simulink model "EPT"  (R2019b)
settings: Solver=FixedStepDiscrete  StartTime=0.0  StopTime=5  FixedStep=0.005  RelTol=1e-3  EnableMultiTasking=on
PreLoadFcn:
  | try, model_open; catch, disp('Error occurred while executing model pre-load callback: model_open.m'); disp('Please assure that the MATLAB working directory is set to the model directory before opening.'); end
InitFcn:
  | try, model_open; catch, end
undefined symbols (not defined in the file or in its folder): Bridge, GCM, H, ln, raptor_get_param_eval, raptor_get_safe_string, raptor_xcp_function
libraries: Raptor_lib x2810, simulink x374, hdlsllib x19
(part 36 of 45)

== system EPT/Foreground_TimeBase_5ms/E//W /BP-OBU_E//W/BP-OBU_E//W/BP-OBU_Warning//Fault_G5/Latch43 ==
  Latch : Inport
  Reset : Inport  Port=2
  Switch1 : Switch  Criteria=u2 > Threshold
  Switch3 : Switch  Criteria=u2 > Threshold
  Unit Delay1 : UnitDelay  SampleTime=-1  HasFrameUpgradeWarning=on
  Output : Outport  VectorParamsAs1DForOutWhenUnconnected=off
  wires:
  Unit Delay1/1 -> Switch1/3
  Switch3/1 -> Output/1, Unit Delay1/1
  Reset/1 -> Switch3/2
  Latch/1 -> Switch1/1, Switch1/2
  Switch1/1 -> Switch3/3

== system EPT/Foreground_TimeBase_5ms/E//W /BP-OBU_E//W/BP-OBU_E//W/BP-OBU_Warning//Fault_G5/Latch44 ==
  Latch : Inport
  Reset : Inport  Port=2
  Switch1 : Switch  Criteria=u2 > Threshold
  Switch3 : Switch  Criteria=u2 > Threshold
  Unit Delay1 : UnitDelay  SampleTime=-1  HasFrameUpgradeWarning=on
  Output : Outport  VectorParamsAs1DForOutWhenUnconnected=off
  wires:
  Switch1/1 -> Switch3/3
  Latch/1 -> Switch1/2, Switch1/1
  Reset/1 -> Switch3/2
  Switch3/1 -> Unit Delay1/1, Output/1
  Unit Delay1/1 -> Switch1/3

== system EPT/Foreground_TimeBase_5ms/E//W /BP-OBU_E//W/BP-OBU_E//W/BP-OBU_Warning//Fault_G5/Latch45 ==
  Latch : Inport
  Reset : Inport  Port=2
  Switch1 : Switch  Criteria=u2 > Threshold
  Switch3 : Switch  Criteria=u2 > Threshold
  Unit Delay1 : UnitDelay  SampleTime=-1  HasFrameUpgradeWarning=on
  Output : Outport  VectorParamsAs1DForOutWhenUnconnected=off
  wires:
  Unit Delay1/1 -> Switch1/3
  Switch3/1 -> Output/1, Unit Delay1/1
  Reset/1 -> Switch3/2
  Latch/1 -> Switch1/1, Switch1/2
  Switch1/1 -> Switch3/3

== system EPT/Foreground_TimeBase_5ms/E//W /BP-OBU_E//W/BP-OBU_E//W/BP-OBU_Warning//Fault_G5/Latch46 ==
  Latch : Inport
  Reset : Inport  Port=2
  Switch1 : Switch  Criteria=u2 > Threshold
  Switch3 : Switch  Criteria=u2 > Threshold
  Unit Delay1 : UnitDelay  SampleTime=-1  HasFrameUpgradeWarning=on
  Output : Outport  VectorParamsAs1DForOutWhenUnconnected=off
  wires:
  Switch1/1 -> Switch3/3
  Latch/1 -> Switch1/2, Switch1/1
  Reset/1 -> Switch3/2
  Switch3/1 -> Unit Delay1/1, Output/1
  Unit Delay1/1 -> Switch1/3

== system EPT/Foreground_TimeBase_5ms/E//W /BP-OBU_E//W/BP-OBU_E//W/BP-OBU_Warning//Fault_G5/Latch47 ==
  Latch : Inport
  Reset : Inport  Port=2
  Switch1 : Switch  Criteria=u2 > Threshold
  Switch3 : Switch  Criteria=u2 > Threshold
  Unit Delay1 : UnitDelay  SampleTime=-1  HasFrameUpgradeWarning=on
  Output : Outport  VectorParamsAs1DForOutWhenUnconnected=off
  wires:
  Unit Delay1/1 -> Switch1/3
  Switch3/1 -> Output/1, Unit Delay1/1
  Reset/1 -> Switch3/2
  Latch/1 -> Switch1/1, Switch1/2
  Switch1/1 -> Switch3/3

== system EPT/Foreground_TimeBase_5ms/E//W /BP-OBU_E//W/BP-OBU_E//W/BP-OBU_Warning//Fault_G5/Latch48 ==
  Latch : Inport
  Reset : Inport  Port=2
  Switch1 : Switch  Criteria=u2 > Threshold
  Switch3 : Switch  Criteria=u2 > Threshold
  Unit Delay1 : UnitDelay  SampleTime=-1  HasFrameUpgradeWarning=on
  Output : Outport  VectorParamsAs1DForOutWhenUnconnected=off
  wires:
  Switch1/1 -> Switch3/3
  Latch/1 -> Switch1/2, Switch1/1
  Reset/1 -> Switch3/2
  Switch3/1 -> Unit Delay1/1, Output/1
  Unit Delay1/1 -> Switch1/3

== system EPT/Foreground_TimeBase_5ms/E//W /BP-OBU_E//W/BP-OBU_E//W/BP-OBU_Warning//Fault_G5/Latch49 ==
  Latch : Inport
  Reset : Inport  Port=2
  Switch1 : Switch  Criteria=u2 > Threshold
  Switch3 : Switch  Criteria=u2 > Threshold
  Unit Delay1 : UnitDelay  SampleTime=-1  HasFrameUpgradeWarning=on
  Output : Outport  VectorParamsAs1DForOutWhenUnconnected=off
  wires:
  Unit Delay1/1 -> Switch1/3
  Switch3/1 -> Output/1, Unit Delay1/1
  Reset/1 -> Switch3/2
  Latch/1 -> Switch1/1, Switch1/2
  Switch1/1 -> Switch3/3

== system EPT/Foreground_TimeBase_5ms/E//W /CAN_E//W/CAN_Fault/BCU CAN Fault/BCU LifeCycle Fault ==
  note: CMU_All_20ms LifeCycle
  note: CMU_All_200ms LifeCycle
  Reset : Inport
  OBC Work : Inport  Port=2
  If Action Subsystem10 : Subsystem  TreatAsAtomicUnit=on
  If Action Subsystem11 : Subsystem  TreatAsAtomicUnit=on
  If Action Subsystem12 : Subsystem  TreatAsAtomicUnit=on
  If Action Subsystem13 : Subsystem  TreatAsAtomicUnit=on
  If Action Subsystem18 : Subsystem  TreatAsAtomicUnit=on
  If Action Subsystem9 : Subsystem  TreatAsAtomicUnit=on
  Latch10 : Subsystem
  Latch11 : Subsystem
  Latch12 : Subsystem
  Latch13 : Subsystem
  Latch14 : Subsystem
  Latch19 : Subsystem
  raptor_data_def1 : Raptor_lib/Data Storage/raptor_data_def  dataName='LifeCycle_Fault_CMU200B0A2'  initValue=0  dataType=boolean  storage=Volatile (RAM)  calVisible=on  calType=Measurement  calDispType=Number  calEnum={'False', 'True'}  calGain=1.0  calOffset=0  calMin=-inf  calMax=inf  calFormat='-1'  calUnit=''  calHelp=''  calAccess=1  calFunction=raptor_xcp_function(gcb)  calDispHeaders=off  calColHeaders={'Col1' 'Col2' 'Col3'}  calRowHeaders={'Row1' 'Row2' 'Row3'}
      settings: SourceProductName=Raptor
  raptor_data_def2 : Raptor_lib/Data Storage/raptor_data_def  dataName='LifeCycle_Fault_CMU200B1A1'  initValue=0  dataType=boolean  storage=Volatile (RAM)  calVisible=on  calType=Measurement  calDispType=Number  calEnum={'False', 'True'}  calGain=1.0  calOffset=0  calMin=-inf  calMax=inf  calFormat='-1'  calUnit=''  calHelp=''  calAccess=1  calFunction=raptor_xcp_function(gcb)  calDispHeaders=off  calColHeaders={'Col1' 'Col2' 'Col3'}  calRowHeaders={'Row1' 'Row2' 'Row3'}
      settings: SourceProductName=Raptor
  raptor_data_def3 : Raptor_lib/Data Storage/raptor_data_def  dataName='LifeCycle_Fault_CMU200B1A2'  initValue=0  dataType=boolean  storage=Volatile (RAM)  calVisible=on  calType=Measurement  calDispType=Number  calEnum={'False', 'True'}  calGain=1.0  calOffset=0  calMin=-inf  calMax=inf  calFormat='-1'  calUnit=''  calHelp=''  calAccess=1  calFunction=raptor_xcp_function(gcb)  calDispHeaders=off  calColHeaders={'Col1' 'Col2' 'Col3'}  calRowHeaders={'Row1' 'Row2' 'Row3'}
      settings: SourceProductName=Raptor
  raptor_data_def31 : Raptor_lib/Data Storage/raptor_data_def  dataName='Flag_B2_200ms'  initValue=0  dataType=boolean  storage=Volatile (RAM)  calVisible=on  calType=Measurement  calDispType=Number  calEnum={'False', 'True'}  calGain=1.0  calOffset=0  calMin=-inf  calMax=inf  calFormat='-1'  calUnit=''  calHelp=''  calAccess=1  calFunction=raptor_xcp_function(gcb)  calDispHeaders=off  calColHeaders={'Col1' 'Col2' 'Col3'}  calRowHeaders={'Row1' 'Row2' 'Row3'}
      settings: SourceProductName=Raptor
  raptor_data_def39 : Raptor_lib/Data Storage/raptor_data_def  dataName='Flag_B0_B1_20ms'  initValue=0  dataType=boolean  storage=Volatile (RAM)  calVisible=on  calType=Measurement  calDispType=Number  calEnum={'False', 'True'}  calGain=1.0  calOffset=0  calMin=-inf  calMax=inf  calFormat='-1'  calUnit=''  calHelp=''  calAccess=1  calFunction=raptor_xcp_function(gcb)  calDispHeaders=off  calColHeaders={'Col1' 'Col2' 'Col3'}  calRowHeaders={'Row1' 'Row2' 'Row3'}
      settings: SourceProductName=Raptor
  raptor_data_def4 : Raptor_lib/Data Storage/raptor_data_def  dataName='LifeCycle_Fault_CMU200B2A1'  initValue=0  dataType=boolean  storage=Volatile (RAM)  calVisible=on  calType=Measurement  calDispType=Number  calEnum={'False', 'True'}  calGain=1.0  calOffset=0  calMin=-inf  calMax=inf  calFormat='-1'  calUnit=''  calHelp=''  calAccess=1  calFunction=raptor_xcp_function(gcb)  calDispHeaders=off  calColHeaders={'Col1' 'Col2' 'Col3'}  calRowHeaders={'Row1' 'Row2' 'Row3'}
      settings: SourceProductName=Raptor
  raptor_data_def5 : Raptor_lib/Data Storage/raptor_data_def  dataName='LifeCycle_Fault_CMU200B2A2'  initValue=0  dataType=boolean  storage=Volatile (RAM)  calVisible=on  calType=Measurement  calDispType=Number  calEnum={'False', 'True'}  calGain=1.0  calOffset=0  calMin=-inf  calMax=inf  calFormat='-1'  calUnit=''  calHelp=''  calAccess=1  calFunction=raptor_xcp_function(gcb)  calDispHeaders=off  calColHeaders={'Col1' 'Col2' 'Col3'}  calRowHeaders={'Row1' 'Row2' 'Row3'}
      settings: SourceProductName=Raptor
  raptor_data_def8 : Raptor_lib/Data Storage/raptor_data_def  dataName='LifeCycle_Fault_CMU200B0A1'  initValue=0  dataType=boolean  storage=Volatile (RAM)  calVisible=on  calType=Measurement  calDispType=Number  calEnum={'False', 'True'}  calGain=1.0  calOffset=0  calMin=-inf  calMax=inf  calFormat='-1'  calUnit=''  calHelp=''  calAccess=1  calFunction=raptor_xcp_function(gcb)  calDispHeaders=off  calColHeaders={'Col1' 'Col2' 'Col3'}  calRowHeaders={'Row1' 'Row2' 'Row3'}
      settings: SourceProductName=Raptor
  raptor_data_read29 : Raptor_lib/Data Storage/raptor_data_read  dataName='CMU1_B0_RC'  dataShape=Scalar  idxSource=Input  idxRow=1  idxCol=1
      settings: SourceProductName=Raptor
  raptor_data_read32 : Raptor_lib/Data Storage/raptor_data_read  dataName='CMU2_B0_RC'  dataShape=Scalar  idxSource=Input  idxRow=1  idxCol=1
      settings: SourceProductName=Raptor
  raptor_data_read33 : Raptor_lib/Data Storage/raptor_data_read  dataName='CMU1_B1_RC'  dataShape=Scalar  idxSource=Input  idxRow=1  idxCol=1
      settings: SourceProductName=Raptor
  raptor_data_read34 : Raptor_lib/Data Storage/raptor_data_read  dataName='CMU1_B2_RC'  dataShape=Scalar  idxSource=Input  idxRow=1  idxCol=1
      settings: SourceProductName=Raptor
  raptor_data_read35 : Raptor_lib/Data Storage/raptor_data_read  dataName='CMU2_B2_RC'  dataShape=Scalar  idxSource=Input  idxRow=1  idxCol=1
      settings: SourceProductName=Raptor
  raptor_data_read41 : Raptor_lib/Data Storage/raptor_data_read  dataName='CMU2_B1_RC'  dataShape=Scalar  idxSource=Input  idxRow=1  idxCol=1
      settings: SourceProductName=Raptor
  raptor_data_read42 : Raptor_lib/Data Storage/raptor_data_read  dataName='Flag_B0_B1_20ms'  dataShape=Scalar  idxSource=Input  idxRow=1  idxCol=1
      settings: SourceProductName=Raptor
  raptor_data_read43 : Raptor_lib/Data Storage/raptor_data_read  dataName='Flag_B2_200ms'  dataShape=Scalar  idxSource=Input  idxRow=1  idxCol=1
      settings: SourceProductName=Raptor
  raptor_data_write23 : Raptor_lib/Data Storage/raptor_data_write  dataName='LifeCycle_Fault_CMU200B0A1'  dataShape=Scalar  idxSource=Input Port  idxRow=1  idxCol=1
      settings: SourceProductName=Raptor
  raptor_data_write24 : Raptor_lib/Data Storage/raptor_data_write  dataName='LifeCycle_Fault_CMU200B0A2'  dataShape=Scalar  idxSource=Input Port  idxRow=1  idxCol=1
      settings: SourceProductName=Raptor
  raptor_data_write25 : Raptor_lib/Data Storage/raptor_data_write  dataName='LifeCycle_Fault_CMU200B1A1'  dataShape=Scalar  idxSource=Input Port  idxRow=1  idxCol=1
      settings: SourceProductName=Raptor
  raptor_data_write26 : Raptor_lib/Data Storage/raptor_data_write  dataName='LifeCycle_Fault_CMU200B2A1'  dataShape=Scalar  idxSource=Input Port  idxRow=1  idxCol=1
      settings: SourceProductName=Raptor
  raptor_data_write27 : Raptor_lib/Data Storage/raptor_data_write  dataName='LifeCycle_Fault_CMU200B2A2'  dataShape=Scalar  idxSource=Input Port  idxRow=1  idxCol=1
      settings: SourceProductName=Raptor
  raptor_data_write32 : Raptor_lib/Data Storage/raptor_data_write  dataName='LifeCycle_Fault_CMU200B1A2'  dataShape=Scalar  idxSource=Input Port  idxRow=1  idxCol=1
      settings: SourceProductName=Raptor
  wires:
  raptor_data_read41/1 -> If Action Subsystem18/1(LifeCycle)
  Latch11/1(Output) -> raptor_data_write25/1
  Latch10/1(Output) -> raptor_data_write23/1
  If Action Subsystem13/1(Trigger) -> Latch14/1(Latch)
  Latch12/1(Output) -> raptor_data_write24/1
  If Action Subsystem18/1(Trigger) -> Latch19/1(Latch)
  raptor_data_read32/1 -> If Action Subsystem11/1(LifeCycle)
  raptor_data_read29/1 -> If Action Subsystem10/1(LifeCycle)
  If Action Subsystem9/1(Trigger) -> Latch11/1(Latch)
  raptor_data_read33/1 -> If Action Subsystem9/1(LifeCycle)
  raptor_data_read43/1 -> If Action Subsystem13/Enable, If Action Subsystem12/Enable
  Reset/1 -> Latch10/2(Reset), Latch19/2(Reset), Latch13/2(Reset), Latch14/2(Reset), Latch11/2(Reset), Latch12/2(Reset)
  raptor_data_read34/1 -> If Action Subsystem12/1(LifeCycle)
  Latch19/1(Output) -> raptor_data_write32/1
  OBC Work/1 -> If Action Subsystem13/2(CanWork), If Action Subsystem12/2(CanWork), If Action Subsystem18/2(CanWork), If Action Subsystem9/2(CanWork), If Action Subsystem11/2(CanWork), If Action Subsystem10/2(CanWork)
  If Action Subsystem10/1(Trigger) -> Latch10/1(Latch)
  raptor_data_read35/1 -> If Action Subsystem13/1(LifeCycle)
  Latch14/1(Output) -> raptor_data_write27/1
  Latch13/1(Output) -> raptor_data_write26/1
  If Action Subsystem11/1(Trigger) -> Latch12/1(Latch)
  If Action Subsystem12/1(Trigger) -> Latch13/1(Latch)
  raptor_data_read42/1 -> If Action Subsystem10/Enable, If Action Subsystem18/Enable, If Action Subsystem9/Enable, If Action Subsystem11/Enable

== system EPT/Foreground_TimeBase_5ms/E//W /CAN_E//W/CAN_Fault/BCU CAN Fault/Error10 ==
  Condition : Inport
  Reset : Inport  Port=2
  Constant : Constant  Value=boolean('1')
  NOT : Logic  Operator=NOT  IconShape=distinctive  AllPortsSameDT=off  OutDataTypeStr=boolean
  Switch : Switch  Criteria=u2 > Threshold
  Switch12 : Switch  Criteria=u2 > Threshold
  Unit Delay : UnitDelay  SampleTime=-1  HasFrameUpgradeWarning=on
  Error : Outport  VectorParamsAs1DForOutWhenUnconnected=off
  wires:
  Constant/1 -> Switch/1, NOT/1
  Unit Delay/1 -> Switch/3
  Switch/1 -> Switch12/3
  Switch12/1 -> Unit Delay/1, Error/1
  Condition/1 -> Switch/2
  Reset/1 -> Switch12/2
  NOT/1 -> Switch12/1

== system EPT/Foreground_TimeBase_5ms/E//W /CAN_E//W/CAN_Fault/BCU CAN Fault/Error11 ==
  Condition : Inport
  Reset : Inport  Port=2
  Constant : Constant  Value=boolean('1')
  NOT : Logic  Operator=NOT  IconShape=distinctive  AllPortsSameDT=off  OutDataTypeStr=boolean
  Switch : Switch  Criteria=u2 > Threshold
  Switch12 : Switch  Criteria=u2 > Threshold
  Unit Delay : UnitDelay  SampleTime=-1  HasFrameUpgradeWarning=on
  Error : Outport  VectorParamsAs1DForOutWhenUnconnected=off
  wires:
  NOT/1 -> Switch12/1
  Reset/1 -> Switch12/2
  Condition/1 -> Switch/2
  Switch12/1 -> Error/1, Unit Delay/1
  Switch/1 -> Switch12/3
  Unit Delay/1 -> Switch/3
  Constant/1 -> NOT/1, Switch/1

== system EPT/Foreground_TimeBase_5ms/E//W /CAN_E//W/CAN_Fault/BCU CAN Fault/Error12 ==
  Condition : Inport
  Reset : Inport  Port=2
  Constant : Constant  Value=boolean('1')
  NOT : Logic  Operator=NOT  IconShape=distinctive  AllPortsSameDT=off  OutDataTypeStr=boolean
  Switch : Switch  Criteria=u2 > Threshold
  Switch12 : Switch  Criteria=u2 > Threshold
  Unit Delay : UnitDelay  SampleTime=-1  HasFrameUpgradeWarning=on
  Error : Outport  VectorParamsAs1DForOutWhenUnconnected=off
  wires:
  Constant/1 -> Switch/1, NOT/1
  Unit Delay/1 -> Switch/3
  Switch/1 -> Switch12/3
  Switch12/1 -> Unit Delay/1, Error/1
  Condition/1 -> Switch/2
  Reset/1 -> Switch12/2
  NOT/1 -> Switch12/1

== system EPT/Foreground_TimeBase_5ms/E//W /CAN_E//W/CAN_Fault/BCU CAN Fault/Error13 ==
  Condition : Inport
  Reset : Inport  Port=2
  Constant : Constant  Value=boolean('1')
  NOT : Logic  Operator=NOT  IconShape=distinctive  AllPortsSameDT=off  OutDataTypeStr=boolean
  Switch : Switch  Criteria=u2 > Threshold
  Switch12 : Switch  Criteria=u2 > Threshold
  Unit Delay : UnitDelay  SampleTime=-1  HasFrameUpgradeWarning=on
  Error : Outport  VectorParamsAs1DForOutWhenUnconnected=off
  wires:
  NOT/1 -> Switch12/1
  Reset/1 -> Switch12/2
  Condition/1 -> Switch/2
  Switch12/1 -> Error/1, Unit Delay/1
  Switch/1 -> Switch12/3
  Unit Delay/1 -> Switch/3
  Constant/1 -> NOT/1, Switch/1

== system EPT/Foreground_TimeBase_5ms/E//W /CAN_E//W/CAN_Fault/BCU CAN Fault/Error3 ==
  Condition : Inport
  Reset : Inport  Port=2
  Constant : Constant  Value=boolean('1')
  NOT : Logic  Operator=NOT  IconShape=distinctive  AllPortsSameDT=off  OutDataTypeStr=boolean
  Switch : Switch  Criteria=u2 > Threshold
  Switch12 : Switch  Criteria=u2 > Threshold
  Unit Delay : UnitDelay  SampleTime=-1  HasFrameUpgradeWarning=on
  Error : Outport  VectorParamsAs1DForOutWhenUnconnected=off
  wires:
  NOT/1 -> Switch12/1
  Reset/1 -> Switch12/2
  Condition/1 -> Switch/2
  Switch12/1 -> Error/1, Unit Delay/1
  Switch/1 -> Switch12/3
  Unit Delay/1 -> Switch/3
  Constant/1 -> NOT/1, Switch/1

== system EPT/Foreground_TimeBase_5ms/E//W /CAN_E//W/CAN_Fault/BCU CAN Fault/Error4 ==
  Condition : Inport
  Reset : Inport  Port=2
  Constant : Constant  Value=boolean('1')
  NOT : Logic  Operator=NOT  IconShape=distinctive  AllPortsSameDT=off  OutDataTypeStr=boolean
  Switch : Switch  Criteria=u2 > Threshold
  Switch12 : Switch  Criteria=u2 > Threshold
  Unit Delay : UnitDelay  SampleTime=-1  HasFrameUpgradeWarning=on
  Error : Outport  VectorParamsAs1DForOutWhenUnconnected=off
  wires:
  Constant/1 -> Switch/1, NOT/1
  Unit Delay/1 -> Switch/3
  Switch/1 -> Switch12/3
  Switch12/1 -> Unit Delay/1, Error/1
  Condition/1 -> Switch/2
  Reset/1 -> Switch12/2
  NOT/1 -> Switch12/1

== system EPT/Foreground_TimeBase_5ms/E//W /CAN_E//W/CAN_Fault/BCU CAN Fault/Error6 ==
  Condition : Inport
  Reset : Inport  Port=2
  Constant : Constant  Value=boolean('1')
  NOT : Logic  Operator=NOT  IconShape=distinctive  AllPortsSameDT=off  OutDataTypeStr=boolean
  Switch : Switch  Criteria=u2 > Threshold
  Switch12 : Switch  Criteria=u2 > Threshold
  Unit Delay : UnitDelay  SampleTime=-1  HasFrameUpgradeWarning=on
  Error : Outport  VectorParamsAs1DForOutWhenUnconnected=off
  wires:
  NOT/1 -> Switch12/1
  Reset/1 -> Switch12/2
  Condition/1 -> Switch/2
  Switch12/1 -> Error/1, Unit Delay/1
  Switch/1 -> Switch12/3
  Unit Delay/1 -> Switch/3
  Constant/1 -> NOT/1, Switch/1

== system EPT/Foreground_TimeBase_5ms/E//W /CAN_E//W/CAN_Fault/BCU CAN Fault/Error7 ==
  Condition : Inport
  Reset : Inport  Port=2
  Constant : Constant  Value=boolean('1')
  NOT : Logic  Operator=NOT  IconShape=distinctive  AllPortsSameDT=off  OutDataTypeStr=boolean
  Switch : Switch  Criteria=u2 > Threshold
  Switch12 : Switch  Criteria=u2 > Threshold
  Unit Delay : UnitDelay  SampleTime=-1  HasFrameUpgradeWarning=on
  Error : Outport  VectorParamsAs1DForOutWhenUnconnected=off
  wires:
  Constant/1 -> Switch/1, NOT/1
  Unit Delay/1 -> Switch/3
  Switch/1 -> Switch12/3
  Switch12/1 -> Unit Delay/1, Error/1
  Condition/1 -> Switch/2
  Reset/1 -> Switch12/2
  NOT/1 -> Switch12/1

== system EPT/Foreground_TimeBase_5ms/E//W /CAN_E//W/CAN_Fault/BCU CAN Fault/Error8 ==
  Condition : Inport
  Reset : Inport  Port=2
  Constant : Constant  Value=boolean('1')
  NOT : Logic  Operator=NOT  IconShape=distinctive  AllPortsSameDT=off  OutDataTypeStr=boolean
  Switch : Switch  Criteria=u2 > Threshold
  Switch12 : Switch  Criteria=u2 > Threshold
  Unit Delay : UnitDelay  SampleTime=-1  HasFrameUpgradeWarning=on
  Error : Outport  VectorParamsAs1DForOutWhenUnconnected=off
  wires:
  NOT/1 -> Switch12/1
  Reset/1 -> Switch12/2
  Condition/1 -> Switch/2
  Switch12/1 -> Error/1, Unit Delay/1
  Switch/1 -> Switch12/3
  Unit Delay/1 -> Switch/3
  Constant/1 -> NOT/1, Switch/1

== system EPT/Foreground_TimeBase_5ms/E//W /CAN_E//W/CAN_Fault/BCU CAN Fault/Error9 ==
  Condition : Inport
  Reset : Inport  Port=2
  Constant : Constant  Value=boolean('1')
  NOT : Logic  Operator=NOT  IconShape=distinctive  AllPortsSameDT=off  OutDataTypeStr=boolean
  Switch : Switch  Criteria=u2 > Threshold
  Switch12 : Switch  Criteria=u2 > Threshold
  Unit Delay : UnitDelay  SampleTime=-1  HasFrameUpgradeWarning=on
  Error : Outport  VectorParamsAs1DForOutWhenUnconnected=off
  wires:
  Constant/1 -> Switch/1, NOT/1
  Unit Delay/1 -> Switch/3
  Switch/1 -> Switch12/3
  Switch12/1 -> Unit Delay/1, Error/1
  Condition/1 -> Switch/2
  Reset/1 -> Switch12/2
  NOT/1 -> Switch12/1

== system EPT/Foreground_TimeBase_5ms/E//W /CAN_E//W/CAN_Fault/BCU CAN Fault/Latch1 ==
  Latch : Inport
  Reset : Inport  Port=2
  Switch1 : Switch  Criteria=u2 > Threshold
  Switch3 : Switch  Criteria=u2 > Threshold
  Unit Delay1 : UnitDelay  SampleTime=-1  HasFrameUpgradeWarning=on
  Output : Outport  VectorParamsAs1DForOutWhenUnconnected=off
  wires:
  Unit Delay1/1 -> Switch1/3
  Switch3/1 -> Output/1, Unit Delay1/1
  Reset/1 -> Switch3/2
  Latch/1 -> Switch1/1, Switch1/2
  Switch1/1 -> Switch3/3

== system EPT/Foreground_TimeBase_5ms/E//W /CAN_E//W/CAN_Fault/BCU CAN Fault/deBounce 12 ==
  >= : Inport
  TimeCount1 : Inport  Port=2
  Constant10 : Constant
  Constant11 : Constant  Value=0
  Constant8 : Constant  Value=0
  CycleTrigger1 : Subsystem
  Switch2 : Switch  Threshold=1
  Switch3 : Switch  Threshold=1
  Unit Delay2 : UnitDelay  SampleTime=-1  HasFrameUpgradeWarning=on
  Tirgger1 : Outport  VectorParamsAs1DForOutWhenUnconnected=off
  wires:
  Constant11/1 -> Switch3/3
  Switch2/1 -> Switch3/1
  Switch3/1 -> CycleTrigger1/1(In1)
  Constant10/1 -> Switch2/3
  Unit Delay2/1 -> Switch2/2
  Constant8/1 -> Switch2/1
  CycleTrigger1/1(Trigger) -> Tirgger1/1, Unit Delay2/1
  >=/1 -> Switch3/2
  TimeCount1/1 -> CycleTrigger1/2(In2)

== system EPT/Foreground_TimeBase_5ms/E//W /CAN_E//W/CAN_Fault/BCU CAN Fault/deBounce 13 ==
  >= : Inport
  TimeCount1 : Inport  Port=2
  Constant10 : Constant
  Constant11 : Constant  Value=0
  Constant8 : Constant  Value=0
  CycleTrigger1 : Subsystem
  Switch2 : Switch  Threshold=1
  Switch3 : Switch  Threshold=1
  Unit Delay2 : UnitDelay  SampleTime=-1  HasFrameUpgradeWarning=on
  Tirgger1 : Outport  VectorParamsAs1DForOutWhenUnconnected=off
  wires:
  TimeCount1/1 -> CycleTrigger1/2(In2)
  >=/1 -> Switch3/2
  CycleTrigger1/1(Trigger) -> Unit Delay2/1, Tirgger1/1
  Constant8/1 -> Switch2/1
  Unit Delay2/1 -> Switch2/2
  Constant10/1 -> Switch2/3
  Switch3/1 -> CycleTrigger1/1(In1)
  Switch2/1 -> Switch3/1
  Constant11/1 -> Switch3/3

== system EPT/Foreground_TimeBase_5ms/E//W /CAN_E//W/CAN_Fault/BCU CAN Fault/deBounce 14 ==
  >= : Inport
  TimeCount1 : Inport  Port=2
  Constant10 : Constant
  Constant11 : Constant  Value=0
  Constant8 : Constant  Value=0
  CycleTrigger1 : Subsystem
  Switch2 : Switch  Threshold=1
  Switch3 : Switch  Threshold=1
  Unit Delay2 : UnitDelay  SampleTime=-1  HasFrameUpgradeWarning=on
  Tirgger1 : Outport  VectorParamsAs1DForOutWhenUnconnected=off
  wires:
  Constant11/1 -> Switch3/3
  Switch2/1 -> Switch3/1
  Switch3/1 -> CycleTrigger1/1(In1)
  Constant10/1 -> Switch2/3
  Unit Delay2/1 -> Switch2/2
  Constant8/1 -> Switch2/1
  CycleTrigger1/1(Trigger) -> Tirgger1/1, Unit Delay2/1
  >=/1 -> Switch3/2
  TimeCount1/1 -> CycleTrigger1/2(In2)

== system EPT/Foreground_TimeBase_5ms/E//W /CAN_E//W/CAN_Fault/BCU CAN Fault/deBounce 15 ==
  >= : Inport
  TimeCount1 : Inport  Port=2
  Constant10 : Constant
  Constant11 : Constant  Value=0
  Constant8 : Constant  Value=0
  CycleTrigger1 : Subsystem
  Switch2 : Switch  Threshold=1
  Switch3 : Switch  Threshold=1
  Unit Delay2 : UnitDelay  SampleTime=-1  HasFrameUpgradeWarning=on
  Tirgger1 : Outport  VectorParamsAs1DForOutWhenUnconnected=off
  wires:
  TimeCount1/1 -> CycleTrigger1/2(In2)
  >=/1 -> Switch3/2
  CycleTrigger1/1(Trigger) -> Unit Delay2/1, Tirgger1/1
  Constant8/1 -> Switch2/1
  Unit Delay2/1 -> Switch2/2
  Constant10/1 -> Switch2/3
  Switch3/1 -> CycleTrigger1/1(In1)
  Switch2/1 -> Switch3/1
  Constant11/1 -> Switch3/3

== system EPT/Foreground_TimeBase_5ms/E//W /CAN_E//W/CAN_Fault/BCU CAN Fault/deBounce 16 ==
  >= : Inport
  TimeCount1 : Inport  Port=2
  Constant10 : Constant
  Constant11 : Constant  Value=0
  Constant8 : Constant  Value=0
  CycleTrigger1 : Subsystem
  Switch2 : Switch  Threshold=1
  Switch3 : Switch  Threshold=1
  Unit Delay2 : UnitDelay  SampleTime=-1  HasFrameUpgradeWarning=on
  Tirgger1 : Outport  VectorParamsAs1DForOutWhenUnconnected=off
  wires:
  Constant11/1 -> Switch3/3
  Switch2/1 -> Switch3/1
  Switch3/1 -> CycleTrigger1/1(In1)
  Constant10/1 -> Switch2/3
  Unit Delay2/1 -> Switch2/2
  Constant8/1 -> Switch2/1
  CycleTrigger1/1(Trigger) -> Tirgger1/1, Unit Delay2/1
  >=/1 -> Switch3/2
  TimeCount1/1 -> CycleTrigger1/2(In2)

== system EPT/Foreground_TimeBase_5ms/E//W /CAN_E//W/CAN_Fault/BCU CAN Fault/deBounce 4 ==
  >= : Inport
  TimeCount1 : Inport  Port=2
  Constant10 : Constant
  Constant11 : Constant  Value=0
  Constant8 : Constant  Value=0
  CycleTrigger1 : Subsystem
  Switch2 : Switch  Threshold=1
  Switch3 : Switch  Threshold=1
  Unit Delay2 : UnitDelay  SampleTime=-1  HasFrameUpgradeWarning=on
  Tirgger1 : Outport  VectorParamsAs1DForOutWhenUnconnected=off
  wires:
  TimeCount1/1 -> CycleTrigger1/2(In2)
  >=/1 -> Switch3/2
  CycleTrigger1/1(Trigger) -> Unit Delay2/1, Tirgger1/1
  Constant8/1 -> Switch2/1
  Unit Delay2/1 -> Switch2/2
  Constant10/1 -> Switch2/3
  Switch3/1 -> CycleTrigger1/1(In1)
  Switch2/1 -> Switch3/1
  Constant11/1 -> Switch3/3

== system EPT/Foreground_TimeBase_5ms/E//W /CAN_E//W/CAN_Fault/BCU CAN Fault/deBounce 5 ==
  >= : Inport
  TimeCount1 : Inport  Port=2
  Constant10 : Constant
  Constant11 : Constant  Value=0
  Constant8 : Constant  Value=0
  CycleTrigger1 : Subsystem
  Switch2 : Switch  Threshold=1
  Switch3 : Switch  Threshold=1
  Unit Delay2 : UnitDelay  SampleTime=-1  HasFrameUpgradeWarning=on
  Tirgger1 : Outport  VectorParamsAs1DForOutWhenUnconnected=off
  wires:
  Constant11/1 -> Switch3/3
  Switch2/1 -> Switch3/1
  Switch3/1 -> CycleTrigger1/1(In1)
  Constant10/1 -> Switch2/3
  Unit Delay2/1 -> Switch2/2
  Constant8/1 -> Switch2/1
  CycleTrigger1/1(Trigger) -> Tirgger1/1, Unit Delay2/1
  >=/1 -> Switch3/2
  TimeCount1/1 -> CycleTrigger1/2(In2)

== system EPT/Foreground_TimeBase_5ms/E//W /CAN_E//W/CAN_Fault/BCU CAN Fault/deBounce 6 ==
  >= : Inport
  TimeCount1 : Inport  Port=2
  Constant10 : Constant
  Constant11 : Constant  Value=0
  Constant8 : Constant  Value=0
  CycleTrigger1 : Subsystem
  Switch2 : Switch  Threshold=1
  Switch3 : Switch  Threshold=1
  Unit Delay2 : UnitDelay  SampleTime=-1  HasFrameUpgradeWarning=on
  Tirgger1 : Outport  VectorParamsAs1DForOutWhenUnconnected=off
  wires:
  TimeCount1/1 -> CycleTrigger1/2(In2)
  >=/1 -> Switch3/2
  CycleTrigger1/1(Trigger) -> Unit Delay2/1, Tirgger1/1
  Constant8/1 -> Switch2/1
  Unit Delay2/1 -> Switch2/2
  Constant10/1 -> Switch2/3
  Switch3/1 -> CycleTrigger1/1(In1)
  Switch2/1 -> Switch3/1
  Constant11/1 -> Switch3/3

== system EPT/Foreground_TimeBase_5ms/E//W /CAN_E//W/CAN_Fault/BCU CAN Fault/deBounce 7 ==
  >= : Inport
  TimeCount1 : Inport  Port=2
  Constant10 : Constant
  Constant11 : Constant  Value=0
  Constant8 : Constant  Value=0
  CycleTrigger1 : Subsystem
  Switch2 : Switch  Threshold=1
  Switch3 : Switch  Threshold=1
  Unit Delay2 : UnitDelay  SampleTime=-1  HasFrameUpgradeWarning=on
  Tirgger1 : Outport  VectorParamsAs1DForOutWhenUnconnected=off
  wires:
  Constant11/1 -> Switch3/3
  Switch2/1 -> Switch3/1
  Switch3/1 -> CycleTrigger1/1(In1)
  Constant10/1 -> Switch2/3
  Unit Delay2/1 -> Switch2/2
  Constant8/1 -> Switch2/1
  CycleTrigger1/1(Trigger) -> Tirgger1/1, Unit Delay2/1
  >=/1 -> Switch3/2
  TimeCount1/1 -> CycleTrigger1/2(In2)

== system EPT/Foreground_TimeBase_5ms/E//W /CAN_E//W/CAN_Fault/BCU CAN Fault/deBounce 8 ==
  >= : Inport
  TimeCount1 : Inport  Port=2
  Constant10 : Constant
  Constant11 : Constant  Value=0
  Constant8 : Constant  Value=0
  CycleTrigger1 : Subsystem
  Switch2 : Switch  Threshold=1
  Switch3 : Switch  Threshold=1
  Unit Delay2 : UnitDelay  SampleTime=-1  HasFrameUpgradeWarning=on
  Tirgger1 : Outport  VectorParamsAs1DForOutWhenUnconnected=off
  wires:
  TimeCount1/1 -> CycleTrigger1/2(In2)
  >=/1 -> Switch3/2
  CycleTrigger1/1(Trigger) -> Unit Delay2/1, Tirgger1/1
  Constant8/1 -> Switch2/1
  Unit Delay2/1 -> Switch2/2
  Constant10/1 -> Switch2/3
  Switch3/1 -> CycleTrigger1/1(In1)
  Switch2/1 -> Switch3/1
  Constant11/1 -> Switch3/3

== system EPT/Foreground_TimeBase_5ms/E//W /CAN_E//W/CAN_Fault/BCU CAN Fault/deBounce 9 ==
  >= : Inport
  TimeCount1 : Inport  Port=2
  Constant10 : Constant
  Constant11 : Constant  Value=0
  Constant8 : Constant  Value=0
  CycleTrigger1 : Subsystem
  Switch2 : Switch  Threshold=1
  Switch3 : Switch  Threshold=1
  Unit Delay2 : UnitDelay  SampleTime=-1  HasFrameUpgradeWarning=on
  Tirgger1 : Outport  VectorParamsAs1DForOutWhenUnconnected=off
  wires:
  Constant11/1 -> Switch3/3
  Switch2/1 -> Switch3/1
  Switch3/1 -> CycleTrigger1/1(In1)
  Constant10/1 -> Switch2/3
  Unit Delay2/1 -> Switch2/2
  Constant8/1 -> Switch2/1
  CycleTrigger1/1(Trigger) -> Tirgger1/1, Unit Delay2/1
  >=/1 -> Switch3/2
  TimeCount1/1 -> CycleTrigger1/2(In2)

== system EPT/Foreground_TimeBase_5ms/E//W /CAN_E//W/CAN_Fault/DCDC CAN Fault/Latch1 ==
  Latch : Inport
  Reset : Inport  Port=2
  Switch1 : Switch  Criteria=u2 > Threshold
  Switch3 : Switch  Criteria=u2 > Threshold
  Unit Delay1 : UnitDelay  SampleTime=-1  HasFrameUpgradeWarning=on
  Output : Outport  VectorParamsAs1DForOutWhenUnconnected=off
  wires:
  Switch1/1 -> Switch3/3
  Latch/1 -> Switch1/2, Switch1/1
  Reset/1 -> Switch3/2
  Switch3/1 -> Unit Delay1/1, Output/1
  Unit Delay1/1 -> Switch1/3

== system EPT/Foreground_TimeBase_5ms/E//W /CAN_E//W/CAN_Fault/DCDC CAN Fault/Latch2 ==
  Latch : Inport
  Reset : Inport  Port=2
  Switch1 : Switch  Criteria=u2 > Threshold
  Switch3 : Switch  Criteria=u2 > Threshold
  Unit Delay1 : UnitDelay  SampleTime=-1  HasFrameUpgradeWarning=on
  Output : Outport  VectorParamsAs1DForOutWhenUnconnected=off
  wires:
  Unit Delay1/1 -> Switch1/3
  Switch3/1 -> Output/1, Unit Delay1/1
  Reset/1 -> Switch3/2
  Latch/1 -> Switch1/1, Switch1/2
  Switch1/1 -> Switch3/3

== system EPT/Foreground_TimeBase_5ms/E//W /CAN_E//W/CAN_Fault/DCDC CAN Fault/deBounce 1 ==
  >= : Inport
  TimeCount1 : Inport  Port=2
  Constant10 : Constant
  Constant11 : Constant  Value=0
  Constant8 : Constant  Value=0
  CycleTrigger1 : Subsystem
  Switch2 : Switch  Threshold=1
  Switch3 : Switch  Threshold=1
  Unit Delay2 : UnitDelay  SampleTime=-1  HasFrameUpgradeWarning=on
  Tirgger1 : Outport  VectorParamsAs1DForOutWhenUnconnected=off
  wires:
  TimeCount1/1 -> CycleTrigger1/2(In2)
  >=/1 -> Switch3/2
  CycleTrigger1/1(Trigger) -> Unit Delay2/1, Tirgger1/1
  Constant8/1 -> Switch2/1
  Unit Delay2/1 -> Switch2/2
  Constant10/1 -> Switch2/3
  Switch3/1 -> CycleTrigger1/1(In1)
  Switch2/1 -> Switch3/1
  Constant11/1 -> Switch3/3

== system EPT/Foreground_TimeBase_5ms/E//W /CAN_E//W/CAN_Fault/DCDC CAN Fault/deBounce 10 ==
  >= : Inport
  TimeCount1 : Inport  Port=2
  Constant10 : Constant
  Constant11 : Constant  Value=0
  Constant8 : Constant  Value=0
  CycleTrigger1 : Subsystem
  Switch2 : Switch  Threshold=1
  Switch3 : Switch  Threshold=1
  Unit Delay2 : UnitDelay  SampleTime=-1  HasFrameUpgradeWarning=on
  Tirgger1 : Outport  VectorParamsAs1DForOutWhenUnconnected=off
  wires:
  Constant11/1 -> Switch3/3
  Switch2/1 -> Switch3/1
  Switch3/1 -> CycleTrigger1/1(In1)
  Constant10/1 -> Switch2/3
  Unit Delay2/1 -> Switch2/2
  Constant8/1 -> Switch2/1
  CycleTrigger1/1(Trigger) -> Tirgger1/1, Unit Delay2/1
  >=/1 -> Switch3/2
  TimeCount1/1 -> CycleTrigger1/2(In2)

== system EPT/Foreground_TimeBase_5ms/E//W /CAN_E//W/CAN_Fault/ECHS CAN Fault/Latch1 ==
  Latch : Inport
  Reset : Inport  Port=2
  Switch1 : Switch  Criteria=u2 > Threshold
  Switch3 : Switch  Criteria=u2 > Threshold
  Unit Delay1 : UnitDelay  SampleTime=-1  HasFrameUpgradeWarning=on
  Output : Outport  VectorParamsAs1DForOutWhenUnconnected=off
  wires:
  Unit Delay1/1 -> Switch1/3
  Switch3/1 -> Output/1, Unit Delay1/1
  Reset/1 -> Switch3/2
  Latch/1 -> Switch1/1, Switch1/2
  Switch1/1 -> Switch3/3

== system EPT/Foreground_TimeBase_5ms/E//W /CAN_E//W/CAN_Fault/ECHS CAN Fault/Latch5 ==
  Latch : Inport
  Reset : Inport  Port=2
  Switch1 : Switch  Criteria=u2 > Threshold
  Switch3 : Switch  Criteria=u2 > Threshold
  Unit Delay1 : UnitDelay  SampleTime=-1  HasFrameUpgradeWarning=on
  Output : Outport  VectorParamsAs1DForOutWhenUnconnected=off
  wires:
  Switch1/1 -> Switch3/3
  Latch/1 -> Switch1/2, Switch1/1
  Reset/1 -> Switch3/2
  Switch3/1 -> Unit Delay1/1, Output/1
  Unit Delay1/1 -> Switch1/3

== system EPT/Foreground_TimeBase_5ms/E//W /CAN_E//W/CAN_Fault/ECHS CAN Fault/deBounce  ==
  >= : Inport
  TimeCount1 : Inport  Port=2
  Constant10 : Constant
  Constant11 : Constant  Value=0
  Constant8 : Constant  Value=0
  CycleTrigger1 : Subsystem
  Switch2 : Switch  Threshold=1
  Switch3 : Switch  Threshold=1
  Unit Delay2 : UnitDelay  SampleTime=-1  HasFrameUpgradeWarning=on
  Tirgger1 : Outport  VectorParamsAs1DForOutWhenUnconnected=off
  wires:
  Constant11/1 -> Switch3/3
  Switch2/1 -> Switch3/1
  Switch3/1 -> CycleTrigger1/1(In1)
  Constant10/1 -> Switch2/3
  Unit Delay2/1 -> Switch2/2
  Constant8/1 -> Switch2/1
  CycleTrigger1/1(Trigger) -> Tirgger1/1, Unit Delay2/1
  >=/1 -> Switch3/2
  TimeCount1/1 -> CycleTrigger1/2(In2)

== system EPT/Foreground_TimeBase_5ms/E//W /CAN_E//W/CAN_Fault/ECHS CAN Fault/deBounce 1 ==
  >= : Inport
  TimeCount1 : Inport  Port=2
  Constant10 : Constant
  Constant11 : Constant  Value=0
  Constant8 : Constant  Value=0
  CycleTrigger1 : Subsystem
  Switch2 : Switch  Threshold=1
  Switch3 : Switch  Threshold=1
  Unit Delay2 : UnitDelay  SampleTime=-1  HasFrameUpgradeWarning=on
  Tirgger1 : Outport  VectorParamsAs1DForOutWhenUnconnected=off
  wires:
  TimeCount1/1 -> CycleTrigger1/2(In2)
  >=/1 -> Switch3/2
  CycleTrigger1/1(Trigger) -> Unit Delay2/1, Tirgger1/1
  Constant8/1 -> Switch2/1
  Unit Delay2/1 -> Switch2/2
  Constant10/1 -> Switch2/3
  Switch3/1 -> CycleTrigger1/1(In1)
  Switch2/1 -> Switch3/1
  Constant11/1 -> Switch3/3

== system EPT/Foreground_TimeBase_5ms/E//W /CAN_E//W/CAN_Fault/MCU CAN Fault/Latch1 ==
  Latch : Inport
  Reset : Inport  Port=2
  Switch1 : Switch  Criteria=u2 > Threshold
  Switch3 : Switch  Criteria=u2 > Threshold
  Unit Delay1 : UnitDelay  SampleTime=-1  HasFrameUpgradeWarning=on
  Output : Outport  VectorParamsAs1DForOutWhenUnconnected=off
  wires:
  Unit Delay1/1 -> Switch1/3
  Switch3/1 -> Output/1, Unit Delay1/1
  Reset/1 -> Switch3/2
  Latch/1 -> Switch1/1, Switch1/2
  Switch1/1 -> Switch3/3

== system EPT/Foreground_TimeBase_5ms/E//W /CAN_E//W/CAN_Fault/MCU CAN Fault/Latch2 ==
  Latch : Inport
  Reset : Inport  Port=2
  Switch1 : Switch  Criteria=u2 > Threshold
  Switch3 : Switch  Criteria=u2 > Threshold
  Unit Delay1 : UnitDelay  SampleTime=-1  HasFrameUpgradeWarning=on
  Output : Outport  VectorParamsAs1DForOutWhenUnconnected=off
  wires:
  Switch1/1 -> Switch3/3
  Latch/1 -> Switch1/2, Switch1/1
  Reset/1 -> Switch3/2
  Switch3/1 -> Unit Delay1/1, Output/1
  Unit Delay1/1 -> Switch1/3

== system EPT/Foreground_TimeBase_5ms/E//W /CAN_E//W/CAN_Fault/MCU CAN Fault/Latch3 ==
  Latch : Inport
  Reset : Inport  Port=2
  Switch1 : Switch  Criteria=u2 > Threshold
  Switch3 : Switch  Criteria=u2 > Threshold
  Unit Delay1 : UnitDelay  SampleTime=-1  HasFrameUpgradeWarning=on
  Output : Outport  VectorParamsAs1DForOutWhenUnconnected=off
  wires:
  Unit Delay1/1 -> Switch1/3
  Switch3/1 -> Output/1, Unit Delay1/1
  Reset/1 -> Switch3/2
  Latch/1 -> Switch1/1, Switch1/2
  Switch1/1 -> Switch3/3

== system EPT/Foreground_TimeBase_5ms/E//W /CAN_E//W/CAN_Fault/MCU CAN Fault/Latch4 ==
  Latch : Inport
  Reset : Inport  Port=2
  Switch1 : Switch  Criteria=u2 > Threshold
  Switch3 : Switch  Criteria=u2 > Threshold
  Unit Delay1 : UnitDelay  SampleTime=-1  HasFrameUpgradeWarning=on
  Output : Outport  VectorParamsAs1DForOutWhenUnconnected=off
  wires:
  Switch1/1 -> Switch3/3
  Latch/1 -> Switch1/2, Switch1/1
  Reset/1 -> Switch3/2
  Switch3/1 -> Unit Delay1/1, Output/1
  Unit Delay1/1 -> Switch1/3

== system EPT/Foreground_TimeBase_5ms/E//W /CAN_E//W/CAN_Fault/MCU CAN Fault/deBounce 1 ==
  >= : Inport
  TimeCount1 : Inport  Port=2
  Constant10 : Constant
  Constant11 : Constant  Value=0
  Constant8 : Constant  Value=0
  CycleTrigger1 : Subsystem
  Switch2 : Switch  Threshold=1
  Switch3 : Switch  Threshold=1
  Unit Delay2 : UnitDelay  SampleTime=-1  HasFrameUpgradeWarning=on
  Tirgger1 : Outport  VectorParamsAs1DForOutWhenUnconnected=off
  wires:
  Constant11/1 -> Switch3/3
  Switch2/1 -> Switch3/1
  Switch3/1 -> CycleTrigger1/1(In1)
  Constant10/1 -> Switch2/3
  Unit Delay2/1 -> Switch2/2
  Constant8/1 -> Switch2/1
  CycleTrigger1/1(Trigger) -> Tirgger1/1, Unit Delay2/1
  >=/1 -> Switch3/2
  TimeCount1/1 -> CycleTrigger1/2(In2)

== system EPT/Foreground_TimeBase_5ms/E//W /CAN_E//W/CAN_Fault/MCU CAN Fault/deBounce 10 ==
  >= : Inport
  TimeCount1 : Inport  Port=2
  Constant10 : Constant
  Constant11 : Constant  Value=0
  Constant8 : Constant  Value=0
  CycleTrigger1 : Subsystem
  Switch2 : Switch  Threshold=1
  Switch3 : Switch  Threshold=1
  Unit Delay2 : UnitDelay  SampleTime=-1  HasFrameUpgradeWarning=on
  Tirgger1 : Outport  VectorParamsAs1DForOutWhenUnconnected=off
  wires:
  TimeCount1/1 -> CycleTrigger1/2(In2)
  >=/1 -> Switch3/2
  CycleTrigger1/1(Trigger) -> Unit Delay2/1, Tirgger1/1
  Constant8/1 -> Switch2/1
  Unit Delay2/1 -> Switch2/2
  Constant10/1 -> Switch2/3
  Switch3/1 -> CycleTrigger1/1(In1)
  Switch2/1 -> Switch3/1
  Constant11/1 -> Switch3/3

== system EPT/Foreground_TimeBase_5ms/E//W /CAN_E//W/CAN_Fault/MCU CAN Fault/deBounce 2 ==
  >= : Inport
  TimeCount1 : Inport  Port=2
  Constant10 : Constant
  Constant11 : Constant  Value=0
  Constant8 : Constant  Value=0
  CycleTrigger1 : Subsystem
  Switch2 : Switch  Threshold=1
  Switch3 : Switch  Threshold=1
  Unit Delay2 : UnitDelay  SampleTime=-1  HasFrameUpgradeWarning=on
  Tirgger1 : Outport  VectorParamsAs1DForOutWhenUnconnected=off
  wires:
  TimeCount1/1 -> CycleTrigger1/2(In2)
  >=/1 -> Switch3/2
  CycleTrigger1/1(Trigger) -> Unit Delay2/1, Tirgger1/1
  Constant8/1 -> Switch2/1
  Unit Delay2/1 -> Switch2/2
  Constant10/1 -> Switch2/3
  Switch3/1 -> CycleTrigger1/1(In1)
  Switch2/1 -> Switch3/1
  Constant11/1 -> Switch3/3

== system EPT/Foreground_TimeBase_5ms/E//W /CAN_E//W/CAN_Fault/MCU CAN Fault/deBounce 3 ==
  >= : Inport
  TimeCount1 : Inport  Port=2
  Constant10 : Constant
  Constant11 : Constant  Value=0
  Constant8 : Constant  Value=0
  CycleTrigger1 : Subsystem
  Switch2 : Switch  Threshold=1
  Switch3 : Switch  Threshold=1
  Unit Delay2 : UnitDelay  SampleTime=-1  HasFrameUpgradeWarning=on
  Tirgger1 : Outport  VectorParamsAs1DForOutWhenUnconnected=off
  wires:
  Constant11/1 -> Switch3/3
  Switch2/1 -> Switch3/1
  Switch3/1 -> CycleTrigger1/1(In1)
  Constant10/1 -> Switch2/3
  Unit Delay2/1 -> Switch2/2
  Constant8/1 -> Switch2/1
  CycleTrigger1/1(Trigger) -> Tirgger1/1, Unit Delay2/1
  >=/1 -> Switch3/2
  TimeCount1/1 -> CycleTrigger1/2(In2)

== system EPT/Foreground_TimeBase_5ms/E//W /CAN_E//W/CAN_Fault/OBC CAN Fault/Latch1 ==
  Latch : Inport
  Reset : Inport  Port=2
  Switch1 : Switch  Criteria=u2 > Threshold
  Switch3 : Switch  Criteria=u2 > Threshold
  Unit Delay1 : UnitDelay  SampleTime=-1  HasFrameUpgradeWarning=on
  Output : Outport  VectorParamsAs1DForOutWhenUnconnected=off
  wires:
  Unit Delay1/1 -> Switch1/3
  Switch3/1 -> Output/1, Unit Delay1/1
  Reset/1 -> Switch3/2
  Latch/1 -> Switch1/1, Switch1/2
  Switch1/1 -> Switch3/3

== system EPT/Foreground_TimeBase_5ms/E//W /CAN_E//W/CAN_Fault/OBC CAN Fault/Latch2 ==
  Latch : Inport
  Reset : Inport  Port=2
  Switch1 : Switch  Criteria=u2 > Threshold
  Switch3 : Switch  Criteria=u2 > Threshold
  Unit Delay1 : UnitDelay  SampleTime=-1  HasFrameUpgradeWarning=on
  Output : Outport  VectorParamsAs1DForOutWhenUnconnected=off
  wires:
  Switch1/1 -> Switch3/3
  Latch/1 -> Switch1/2, Switch1/1
  Reset/1 -> Switch3/2
  Switch3/1 -> Unit Delay1/1, Output/1
  Unit Delay1/1 -> Switch1/3

== system EPT/Foreground_TimeBase_5ms/E//W /CAN_E//W/CAN_Fault/OBC CAN Fault/deBounce 1  ==
  >= : Inport
  TimeCount1 : Inport  Port=2
  Constant10 : Constant
  Constant11 : Constant  Value=0
  Constant8 : Constant  Value=0
  CycleTrigger1 : Subsystem
  Switch2 : Switch  Threshold=1
  Switch3 : Switch  Threshold=1
  Unit Delay2 : UnitDelay  SampleTime=-1  HasFrameUpgradeWarning=on
  Tirgger1 : Outport  VectorParamsAs1DForOutWhenUnconnected=off
  wires:
  TimeCount1/1 -> CycleTrigger1/2(In2)
  >=/1 -> Switch3/2
  CycleTrigger1/1(Trigger) -> Unit Delay2/1, Tirgger1/1
  Constant8/1 -> Switch2/1
  Unit Delay2/1 -> Switch2/2
  Constant10/1 -> Switch2/3
  Switch3/1 -> CycleTrigger1/1(In1)
  Switch2/1 -> Switch3/1
  Constant11/1 -> Switch3/3

== system EPT/Foreground_TimeBase_5ms/E//W /CAN_E//W/CAN_Fault/OBC CAN Fault/deBounce 2 ==
  >= : Inport
  TimeCount1 : Inport  Port=2
  Constant10 : Constant
  Constant11 : Constant  Value=0
  Constant8 : Constant  Value=0
  CycleTrigger1 : Subsystem
  Switch2 : Switch  Threshold=1
  Switch3 : Switch  Threshold=1
  Unit Delay2 : UnitDelay  SampleTime=-1  HasFrameUpgradeWarning=on
  Tirgger1 : Outport  VectorParamsAs1DForOutWhenUnconnected=off
  wires:
  Constant11/1 -> Switch3/3
  Switch2/1 -> Switch3/1
  Switch3/1 -> CycleTrigger1/1(In1)
  Constant10/1 -> Switch2/3
  Unit Delay2/1 -> Switch2/2
  Constant8/1 -> Switch2/1
  CycleTrigger1/1(Trigger) -> Tirgger1/1, Unit Delay2/1
  >=/1 -> Switch3/2
  TimeCount1/1 -> CycleTrigger1/2(In2)

== system EPT/Foreground_TimeBase_5ms/System Setup/HV_Setup()/CHG_Mode/CHG Full Flag/Delay ==
  Condition : Inport
  TimeCount : Inport  Port=2
  Constant10 : Constant
  Constant11 : Constant  Value=0
  Constant8 : Constant  Value=0
  CycleTrigger : Subsystem
  Switch2 : Switch  Threshold=1
  Switch3 : Switch  Threshold=1
  Unit Delay1 : UnitDelay  SampleTime=-1  HasFrameUpgradeWarning=on
  Unit Delay2 : UnitDelay  SampleTime=-1  HasFrameUpgradeWarning=on
  Output : Outport  VectorParamsAs1DForOutWhenUnconnected=off
  wires:
  Unit Delay1/1 -> Output/1
  Switch2/1 -> Unit Delay2/1
  Unit Delay2/1 -> Switch3/1
  Constant11/1 -> Switch3/3
  Switch3/1 -> CycleTrigger/1(In1)
  Constant10/1 -> Switch2/3
  Constant8/1 -> Switch2/1
  CycleTrigger/1(Trigger) -> Unit Delay1/1, Switch2/2
  Condition/1 -> Switch3/2
  TimeCount/1 -> CycleTrigger/2(In2)

== system EPT/Foreground_TimeBase_5ms/System Setup/HV_Setup()/CHG_Mode/CHG Full Flag/Latch2 ==
  Latch : Inport
  Reset : Inport  Port=2
  Switch1 : Switch  Criteria=u2 > Threshold
  Switch3 : Switch  Criteria=u2 > Threshold
  Unit Delay1 : UnitDelay  SampleTime=-1  HasFrameUpgradeWarning=on
  Output : Outport  VectorParamsAs1DForOutWhenUnconnected=off
  wires:
  Unit Delay1/1 -> Switch1/3
  Switch3/1 -> Output/1, Unit Delay1/1
  Reset/1 -> Switch3/2
  Latch/1 -> Switch1/1, Switch1/2
  Switch1/1 -> Switch3/3

== system EPT/Foreground_TimeBase_5ms/System Setup/HV_Setup()/CHG_Mode/CHG_Mode_Function/CHG_Mode_Function ==
  Enable : EnablePort  StatesWhenEnabling=reset
  Cmd_CHG_Current_PID : Subsystem  TreatAsAtomicUnit=on
  Constant : Constant  Value=0  OutDataTypeStr=uint8
  Constant1 : Constant  Value=0  OutDataTypeStr=uint8
  OBC Work : Subsystem  TreatAsAtomicUnit=on
  raptor_adjustment1 : Raptor_lib/Data Storage/raptor_adjustment  paramName='Cal_Cmd_CHGV'  nameSource=Parameter  initValue=110  dataType=double  storage=Calibration  calDispType=Number  calEnum={'False', 'True'}  calGain=1.0  calOffset=0.0  calMax=inf  calMin=-inf  calFormat='-1'  calUnit=''  calHelp=''  calAccess=1  calFunction=raptor_xcp_function(gcb)  calDispHeaders=off  calColHeaders={'Col1' 'Col2' 'Col3'}  calRowHeaders={'Row1' 'Row2' 'Row3'}
      settings: SourceProductName=Raptor
  raptor_data_write2 : Raptor_lib/Data Storage/raptor_data_write  dataName='EPT_OBC_EN'  dataShape=Scalar  idxSource=Input Port  idxRow=1  idxCol=1
      settings: SourceProductName=Raptor
  raptor_data_write3 : Raptor_lib/Data Storage/raptor_data_write  dataName='EPT_OBC_STA'  dataShape=Scalar  idxSource=Input Port  idxRow=1  idxCol=1
      settings: SourceProductName=Raptor
  raptor_data_write4 : Raptor_lib/Data Storage/raptor_data_write  dataName='EPT_OBC_VOUT_CMD'  dataShape=Scalar  idxSource=Input Port  idxRow=1  idxCol=1
      settings: SourceProductName=Raptor
  wires:
  raptor_adjustment1/1 -> raptor_data_write4/1
  Constant1/1 -> raptor_data_write3/1
  Constant/1 -> raptor_data_write2/1

== system EPT/Foreground_TimeBase_5ms/System Setup/HV_Setup()/CHG_Mode/CHG_Mode_Function/Delay ==
  Condition : Inport
  TimeCount : Inport  Port=2
  Constant10 : Constant
  Constant11 : Constant  Value=0
  Constant8 : Constant  Value=0
  CycleTrigger : Subsystem
  Switch2 : Switch  Threshold=1
  Switch3 : Switch  Threshold=1
  Unit Delay1 : UnitDelay  SampleTime=-1  HasFrameUpgradeWarning=on
  Unit Delay2 : UnitDelay  SampleTime=-1  HasFrameUpgradeWarning=on
  Output : Outport  VectorParamsAs1DForOutWhenUnconnected=off
  wires:
  TimeCount/1 -> CycleTrigger/2(In2)
  Condition/1 -> Switch3/2
  CycleTrigger/1(Trigger) -> Switch2/2, Unit Delay1/1
  Constant8/1 -> Switch2/1
  Constant10/1 -> Switch2/3
  Switch3/1 -> CycleTrigger/1(In1)
  Constant11/1 -> Switch3/3
  Unit Delay2/1 -> Switch3/1
  Switch2/1 -> Unit Delay2/1
  Unit Delay1/1 -> Output/1

== system EPT/Foreground_TimeBase_5ms/System Setup/HV_Setup()/CHG_Mode/CHG_Mode_Function/Latch ==
  Latch : Inport
  Reset : Inport  Port=2
  Switch1 : Switch  Criteria=u2 > Threshold
  Switch3 : Switch  Criteria=u2 > Threshold
  Unit Delay1 : UnitDelay  SampleTime=-1  HasFrameUpgradeWarning=on
  Output : Outport  VectorParamsAs1DForOutWhenUnconnected=off
  wires:
  Unit Delay1/1 -> Switch1/3
  Switch3/1 -> Output/1, Unit Delay1/1
  Reset/1 -> Switch3/2
  Latch/1 -> Switch1/1, Switch1/2
  Switch1/1 -> Switch3/3

== system EPT/Foreground_TimeBase_5ms/System Setup/HV_Setup()/CHG_Mode/Delay1/CycleTrigger ==
  In1 : Inport
  In2 : Inport  Port=2
  Add : Sum
  Add2 : Sum  Inputs=+-
  Constant2 : Constant  Value=0
  Constant3 : Constant
  Data Type Conversion1 : DataTypeConversion
  Data Type Conversion2 : DataTypeConversion
  Relational Operator1 : RelationalOperator  OutDataTypeStr=boolean  RndMeth=Simplest
  Saturation : Saturate  UpperLimit=inf  LowerLimit=2
  Switch : Switch  Threshold=1
  Unit Delay : UnitDelay  SampleTime=-1  HasFrameUpgradeWarning=on
  Trigger : Outport  VectorParamsAs1DForOutWhenUnconnected=off
  wires:
  Saturation/1 -> Add2/1
  Add/1 -> Switch/1
  In1/1 -> Data Type Conversion2/1
  Unit Delay/1 -> Add/1
  Switch/1 -> Relational Operator1/1, Unit Delay/1
  Relational Operator1/1 -> Trigger/1
  Data Type Conversion1/1 -> Relational Operator1/2
  Constant2/1 -> Switch/3
  Data Type Conversion2/1 -> Add/2, Switch/2
  Add2/1 -> Data Type Conversion1/1
  In2/1 -> Saturation/1
  Constant3/1 -> Add2/2

== system EPT/Foreground_TimeBase_5ms/System Setup/HV_Setup()/CHG_Mode/Disable_CHG_Mode_Function/Delay ==
  Condition : Inport
  TimeCount : Inport  Port=2
  Constant10 : Constant
  Constant11 : Constant  Value=0
  Constant8 : Constant  Value=0
  CycleTrigger : Subsystem
  Switch2 : Switch  Threshold=1
  Switch3 : Switch  Threshold=1
  Unit Delay1 : UnitDelay  SampleTime=-1  HasFrameUpgradeWarning=on
  Unit Delay2 : UnitDelay  SampleTime=-1  HasFrameUpgradeWarning=on
  Output : Outport  VectorParamsAs1DForOutWhenUnconnected=off
  wires:
  TimeCount/1 -> CycleTrigger/2(In2)
  Condition/1 -> Switch3/2
  CycleTrigger/1(Trigger) -> Switch2/2, Unit Delay1/1
  Constant8/1 -> Switch2/1
  Constant10/1 -> Switch2/3
  Switch3/1 -> CycleTrigger/1(In1)
  Constant11/1 -> Switch3/3
  Unit Delay2/1 -> Switch3/1
  Switch2/1 -> Unit Delay2/1
  Unit Delay1/1 -> Output/1

== system EPT/Foreground_TimeBase_5ms/System Setup/HV_Setup()/CHG_Mode/Disable_CHG_Mode_Function/Disable_CHG_Enable ==
  Enable : EnablePort  StatesWhenEnabling=reset
  Constant : Constant  Value=0  OutDataTypeStr=boolean
  raptor_data_write1 : Raptor_lib/Data Storage/raptor_data_write  dataName='A10_CHG_Enable'  dataShape=Scalar  idxSource=Input Port  idxRow=1  idxCol=1
      settings: SourceProductName=Raptor
  wires:
  Constant/1 -> raptor_data_write1/1

== system EPT/Foreground_TimeBase_5ms/System Setup/HV_Setup()/CHG_Mode/Disable_CHG_Mode_Function/Disable_CHG_Mode_Function ==
  Enable : EnablePort  StatesWhenEnabling=reset
  Disable_CHG_Mode_Function : Subsystem
  "OBC Off " : Subsystem  TreatAsAtomicUnit=on

== system EPT/Foreground_TimeBase_5ms/System Setup/HV_Setup()/CHG_Mode/Disable_CHG_Mode_Function/Latch ==
  Latch : Inport
  Reset : Inport  Port=2
  Switch1 : Switch  Criteria=u2 > Threshold
  Switch3 : Switch  Criteria=u2 > Threshold
  Unit Delay1 : UnitDelay  SampleTime=-1  HasFrameUpgradeWarning=on
  Output : Outport  VectorParamsAs1DForOutWhenUnconnected=off
  wires:
  Unit Delay1/1 -> Switch1/3
  Switch3/1 -> Output/1, Unit Delay1/1
  Reset/1 -> Switch3/2
  Latch/1 -> Switch1/1, Switch1/2
  Switch1/1 -> Switch3/3

== system EPT/Foreground_TimeBase_5ms/System Setup/HV_Setup()/Drive_Mode/Disable_Drive_Mode/Delay ==
  Condition : Inport
  TimeCount : Inport  Port=2
  Constant10 : Constant
  Constant11 : Constant  Value=0
  Constant8 : Constant  Value=0
  CycleTrigger : Subsystem
  Switch2 : Switch  Threshold=1
  Switch3 : Switch  Threshold=1
  Unit Delay1 : UnitDelay  SampleTime=-1  HasFrameUpgradeWarning=on
  Unit Delay2 : UnitDelay  SampleTime=-1  HasFrameUpgradeWarning=on
  Output : Outport  VectorParamsAs1DForOutWhenUnconnected=off
  wires:
  TimeCount/1 -> CycleTrigger/2(In2)
  Condition/1 -> Switch3/2
  CycleTrigger/1(Trigger) -> Switch2/2, Unit Delay1/1
  Constant8/1 -> Switch2/1
  Constant10/1 -> Switch2/3
  Switch3/1 -> CycleTrigger/1(In1)
  Constant11/1 -> Switch3/3
  Unit Delay2/1 -> Switch3/1
  Switch2/1 -> Unit Delay2/1
  Unit Delay1/1 -> Output/1
